simulink model "CubeSatTEST"  (R2024b)
settings: Solver=ode4  StartTime=simul.t0  StopTime=simul.tf  FixedStep=0.01  RelTol=1e-3
values from neighbouring files (symbols this model uses):
  alpha1 = 0.7    [mainSimTEST.m]
  alpha2 = 0.3    [mainSimTEST.m]
undefined symbols (not defined in the file or in its folder): act, DiscIntNeverNeededParam, env, flag, IC, K, orb, sat, sens
libraries: matrix_library x55, simulink_extras x5, simulink x2
(part 8 of 10)

== system CubeSatTEST/Real World/Hardware Models/Actuators/CMG + Control Logic/CMG/State/B assembler ==
  beta : Inport
  delta : Inport  Port=2
  Cos : Trigonometry  Operator=cos
  Cos1 : Trigonometry  Operator=cos
  Gain{,1..3} (4 alike) : Gain  Gain=-1
  Matrix Concatenate : Concatenate  NumInputs=4  Mode=Multidimensional array  ConcatenateDimension=2
  Matrix Concatenate{1..4} (4 alike) : Concatenate  NumInputs=3  Mode=Multidimensional array
  Product{,1..7} (8 alike) : Product
  Selector : Selector  InputPortWidth=4  IndexOptions=Index vector (dialog)  Indices=1  OutputSizes=1
  Selector1 : Selector  InputPortWidth=4  IndexOptions=Index vector (dialog)  Indices=1  OutputSizes=1
  Selector10 : Selector  InputPortWidth=4  IndexOptions=Index vector (dialog)  Indices=4  OutputSizes=1
  Selector11 : Selector  InputPortWidth=4  IndexOptions=Index vector (dialog)  Indices=4  OutputSizes=1
  Selector2 : Selector  InputPortWidth=4  IndexOptions=Index vector (dialog)  Indices=1  OutputSizes=1
  Selector3 : Selector  InputPortWidth=4  IndexOptions=Index vector (dialog)  Indices=2  OutputSizes=1
  Selector4 : Selector  InputPortWidth=4  IndexOptions=Index vector (dialog)  Indices=2  OutputSizes=1
  Selector5 : Selector  InputPortWidth=4  IndexOptions=Index vector (dialog)  Indices=2  OutputSizes=1
  Selector6 : Selector  InputPortWidth=4  IndexOptions=Index vector (dialog)  Indices=3  OutputSizes=1
  Selector7 : Selector  InputPortWidth=4  IndexOptions=Index vector (dialog)  Indices=3  OutputSizes=1
  Selector8 : Selector  InputPortWidth=4  IndexOptions=Index vector (dialog)  Indices=3  OutputSizes=1
  Selector9 : Selector  InputPortWidth=4  IndexOptions=Index vector (dialog)  Indices=4  OutputSizes=1
  Sin : Trigonometry
  Sin1 : Trigonometry
  B : Outport
  wires:
  Cos/1 -> [cosd]
  Sin/1 -> [sind]
  delta/1 -> Cos/1, Sin/1
  beta/1 -> Sin1/1, Cos1/1
  Sin1/1 -> [sinb]
  Cos1/1 -> [cosb]
  Gain/1 -> Matrix Concatenate1/1
  Gain1/1 -> Matrix Concatenate1/2
  Gain2/1 -> Matrix Concatenate2/2
  Gain3/1 -> Matrix Concatenate4/1
  Matrix Concatenate1/1 -> Matrix Concatenate/1
  Matrix Concatenate2/1 -> Matrix Concatenate/2
  Matrix Concatenate3/1 -> Matrix Concatenate/3
  Matrix Concatenate4/1 -> Matrix Concatenate/4
  Matrix Concatenate/1 -> B/1
  Product/1 -> Gain/1
  Product1/1 -> Matrix Concatenate1/3
  Product2/1 -> Gain2/1
  Product3/1 -> Matrix Concatenate2/3
  Product4/1 -> Matrix Concatenate3/1
  Product5/1 -> Matrix Concatenate3/3
  Product6/1 -> Matrix Concatenate4/2
  Product7/1 -> Matrix Concatenate4/3
  Selector/1 -> Gain1/1
  Selector1/1 -> Product1/2
  Selector2/1 -> Product/2
  Selector3/1 -> Matrix Concatenate2/1
  Selector4/1 -> Product2/1
  Selector5/1 -> Product3/2
  Selector6/1 -> Product5/2
  Selector7/1 -> Matrix Concatenate3/2
  Selector8/1 -> Product4/1
  Selector9/1 -> Gain3/1
  Selector10/1 -> Product6/2
  Selector11/1 -> Product7/2
  [sind] -> Selector/1
  [sind] -> Selector3/1
  [sind] -> Selector7/1
  [sind] -> Selector9/1
  [cosd] -> Selector2/1
  [cosd] -> Selector1/1
  [cosd] -> Selector5/1
  [cosd] -> Selector4/1
  [cosd] -> Selector8/1
  [cosd] -> Selector6/1
  [cosd] -> Selector11/1
  [cosd] -> Selector10/1
  [cosb] -> Product/1
  [cosb] -> Product2/2
  [cosb] -> Product4/2
  [cosb] -> Product6/1
  [sinb] -> Product1/1
  [sinb] -> Product3/1
  [sinb] -> Product5/1
  [sinb] -> Product7/1

== system CubeSatTEST/OBC/Navigation1/Sequential Rotations/Q method/q_opt computing/Det 3x3/Adj 3x3/C11 ==
  In1 : Inport
  22 : Selector  NumberOfDimensions=2  InputPortWidth=3  IndexOptions=Index vector (dialog),Index vector (dialog)  Indices=2,2  OutputSizes=1,1
  23 : Selector  NumberOfDimensions=2  InputPortWidth=3  IndexOptions=Index vector (dialog),Index vector (dialog)  Indices=2,3  OutputSizes=1,1
  32 : Selector  NumberOfDimensions=2  InputPortWidth=3  IndexOptions=Index vector (dialog),Index vector (dialog)  Indices=3,2  OutputSizes=1,1
  33 : Selector  NumberOfDimensions=2  InputPortWidth=3  IndexOptions=Index vector (dialog),Index vector (dialog)  Indices=3,3  OutputSizes=1,1
  Product : Product
  Product1 : Product
  Subtract : Sum  Inputs=+-
  Out1 : Outport
  wires:
  In1/1 -> 32/1, 23/1, 33/1, 22/1
  22/1 -> Product/1
  33/1 -> Product/2
  23/1 -> Product1/1
  32/1 -> Product1/2
  Subtract/1 -> Out1/1
  Product/1 -> Subtract/1
  Product1/1 -> Subtract/2

== system CubeSatTEST/OBC/Navigation1/Sequential Rotations/Q method/q_opt computing/Det 3x3/Adj 3x3/C12 ==
  In1 : Inport
  21 : Selector  NumberOfDimensions=2  InputPortWidth=3  IndexOptions=Index vector (dialog),Index vector (dialog)  Indices=2,1  OutputSizes=1,1
  23 : Selector  NumberOfDimensions=2  InputPortWidth=3  IndexOptions=Index vector (dialog),Index vector (dialog)  Indices=2,3  OutputSizes=1,1
  31 : Selector  NumberOfDimensions=2  InputPortWidth=3  IndexOptions=Index vector (dialog),Index vector (dialog)  Indices=3,1  OutputSizes=1,1
  33 : Selector  NumberOfDimensions=2  InputPortWidth=3  IndexOptions=Index vector (dialog),Index vector (dialog)  Indices=3,3  OutputSizes=1,1
  Gain : Gain  Gain=-1
  Product : Product
  Product1 : Product
  Subtract : Sum  Inputs=+-
  Out1 : Outport
  wires:
  In1/1 -> 23/1, 31/1, 33/1, 21/1
  21/1 -> Product/1
  33/1 -> Product/2
  31/1 -> Product1/1
  23/1 -> Product1/2
  Subtract/1 -> Gain/1
  Product/1 -> Subtract/1
  Product1/1 -> Subtract/2
  Gain/1 -> Out1/1

== system CubeSatTEST/OBC/Navigation1/Sequential Rotations/Q method/q_opt computing/Det 3x3/Adj 3x3/C13 ==
  In1 : Inport
  21 : Selector  NumberOfDimensions=2  InputPortWidth=3  IndexOptions=Index vector (dialog),Index vector (dialog)  Indices=2,1  OutputSizes=1,1
  22 : Selector  NumberOfDimensions=2  InputPortWidth=3  IndexOptions=Index vector (dialog),Index vector (dialog)  Indices=2,2  OutputSizes=1,1
  31 : Selector  NumberOfDimensions=2  InputPortWidth=3  IndexOptions=Index vector (dialog),Index vector (dialog)  Indices=3,1  OutputSizes=1,1
  32 : Selector  NumberOfDimensions=2  InputPortWidth=3  IndexOptions=Index vector (dialog),Index vector (dialog)  Indices=3,2  OutputSizes=1,1
  Product : Product
  Product1 : Product
  Subtract : Sum  Inputs=+-
  Out1 : Outport
  wires:
  In1/1 -> 31/1, 22/1, 32/1, 21/1
  21/1 -> Product/1
  32/1 -> Product/2
  22/1 -> Product1/1
  31/1 -> Product1/2
  Subtract/1 -> Out1/1
  Product/1 -> Subtract/1
  Product1/1 -> Subtract/2

== system CubeSatTEST/OBC/Navigation1/Sequential Rotations/Q method/q_opt computing/Det 3x3/Adj 3x3/C21 ==
  In1 : Inport
  12 : Selector  NumberOfDimensions=2  InputPortWidth=3  IndexOptions=Index vector (dialog),Index vector (dialog)  Indices=1,2  OutputSizes=1,1
  13 : Selector  NumberOfDimensions=2  InputPortWidth=3  IndexOptions=Index vector (dialog),Index vector (dialog)  Indices=1,3  OutputSizes=1,1
  32 : Selector  NumberOfDimensions=2  InputPortWidth=3  IndexOptions=Index vector (dialog),Index vector (dialog)  Indices=3,2  OutputSizes=1,1
  33 : Selector  NumberOfDimensions=2  InputPortWidth=3  IndexOptions=Index vector (dialog),Index vector (dialog)  Indices=3,3  OutputSizes=1,1
  Gain : Gain  Gain=-1
  Product : Product
  Product1 : Product
  Subtract : Sum  Inputs=+-
  Out1 : Outport
  wires:
  In1/1 -> 32/1, 13/1, 33/1, 12/1
  12/1 -> Product/1
  33/1 -> Product/2
  13/1 -> Product1/1
  32/1 -> Product1/2
  Subtract/1 -> Gain/1
  Product/1 -> Subtract/1
  Product1/1 -> Subtract/2
  Gain/1 -> Out1/1

== system CubeSatTEST/OBC/Navigation1/Sequential Rotations/Q method/q_opt computing/Det 3x3/Adj 3x3/C22 ==
  In1 : Inport
  11 : Selector  NumberOfDimensions=2  InputPortWidth=3  IndexOptions=Index vector (dialog),Index vector (dialog)  Indices=1,1  OutputSizes=1,1
  13 : Selector  NumberOfDimensions=2  InputPortWidth=3  IndexOptions=Index vector (dialog),Index vector (dialog)  Indices=1,3  OutputSizes=1,1
  31 : Selector  NumberOfDimensions=2  InputPortWidth=3  IndexOptions=Index vector (dialog),Index vector (dialog)  Indices=3,1  OutputSizes=1,1
  33 : Selector  NumberOfDimensions=2  InputPortWidth=3  IndexOptions=Index vector (dialog),Index vector (dialog)  Indices=3,3  OutputSizes=1,1
  Product : Product
  Product1 : Product
  Subtract : Sum  Inputs=+-
  Out1 : Outport
  wires:
  In1/1 -> 31/1, 13/1, 33/1, 11/1
  11/1 -> Product/1
  33/1 -> Product/2
  13/1 -> Product1/1
  31/1 -> Product1/2
  Subtract/1 -> Out1/1
  Product/1 -> Subtract/1
  Product1/1 -> Subtract/2

== system CubeSatTEST/OBC/Navigation1/Sequential Rotations/Q method/q_opt computing/Det 3x3/Adj 3x3/C23 ==
  In1 : Inport
  11 : Selector  NumberOfDimensions=2  InputPortWidth=3  IndexOptions=Index vector (dialog),Index vector (dialog)  Indices=1,1  OutputSizes=1,1
  12 : Selector  NumberOfDimensions=2  InputPortWidth=3  IndexOptions=Index vector (dialog),Index vector (dialog)  Indices=1,2  OutputSizes=1,1
  31 : Selector  NumberOfDimensions=2  InputPortWidth=3  IndexOptions=Index vector (dialog),Index vector (dialog)  Indices=3,1  OutputSizes=1,1
  32 : Selector  NumberOfDimensions=2  InputPortWidth=3  IndexOptions=Index vector (dialog),Index vector (dialog)  Indices=3,2  OutputSizes=1,1
  Gain : Gain  Gain=-1
  Product : Product
  Product1 : Product
  Subtract : Sum  Inputs=+-
  Out1 : Outport
  wires:
  In1/1 -> 12/1, 31/1, 32/1, 11/1
  11/1 -> Product/1
  32/1 -> Product/2
  31/1 -> Product1/1
  12/1 -> Product1/2
  Subtract/1 -> Gain/1
  Product/1 -> Subtract/1
  Product1/1 -> Subtract/2
  Gain/1 -> Out1/1

== system CubeSatTEST/OBC/Navigation1/Sequential Rotations/Q method/q_opt computing/Det 3x3/Adj 3x3/C31 ==
  In1 : Inport
  12 : Selector  NumberOfDimensions=2  InputPortWidth=3  IndexOptions=Index vector (dialog),Index vector (dialog)  Indices=1,2  OutputSizes=1,1
  13 : Selector  NumberOfDimensions=2  InputPortWidth=3  IndexOptions=Index vector (dialog),Index vector (dialog)  Indices=1,3  OutputSizes=1,1
  22 : Selector  NumberOfDimensions=2  InputPortWidth=3  IndexOptions=Index vector (dialog),Index vector (dialog)  Indices=2,2  OutputSizes=1,1
  23 : Selector  NumberOfDimensions=2  InputPortWidth=3  IndexOptions=Index vector (dialog),Index vector (dialog)  Indices=2,3  OutputSizes=1,1
  Product : Product
  Product1 : Product
  Subtract : Sum  Inputs=+-
  Out1 : Outport
  wires:
  In1/1 -> 22/1, 13/1, 23/1, 12/1
  12/1 -> Product/1
  23/1 -> Product/2
  13/1 -> Product1/1
  22/1 -> Product1/2
  Subtract/1 -> Out1/1
  Product/1 -> Subtract/1
  Product1/1 -> Subtract/2

== system CubeSatTEST/OBC/Navigation1/Sequential Rotations/Q method/q_opt computing/Det 3x3/Adj 3x3/C32 ==
  In1 : Inport
  11 : Selector  NumberOfDimensions=2  InputPortWidth=3  IndexOptions=Index vector (dialog),Index vector (dialog)  Indices=1,1  OutputSizes=1,1
  13 : Selector  NumberOfDimensions=2  InputPortWidth=3  IndexOptions=Index vector (dialog),Index vector (dialog)  Indices=1,3  OutputSizes=1,1
  23 : Selector  NumberOfDimensions=2  InputPortWidth=3  IndexOptions=Index vector (dialog),Index vector (dialog)  Indices=2,3  OutputSizes=1,1
  31 : Selector  NumberOfDimensions=2  InputPortWidth=3  IndexOptions=Index vector (dialog),Index vector (dialog)  Indices=3,1  OutputSizes=1,1
  Gain : Gain  Gain=-1
  Product : Product
  Product1 : Product
  Subtract : Sum  Inputs=+-
  Out1 : Outport
  wires:
  In1/1 -> 31/1, 13/1, 23/1, 11/1
  11/1 -> Product/1
  23/1 -> Product/2
  13/1 -> Product1/1
  31/1 -> Product1/2
  Subtract/1 -> Gain/1
  Product/1 -> Subtract/1
  Product1/1 -> Subtract/2
  Gain/1 -> Out1/1

== system CubeSatTEST/OBC/Navigation1/Sequential Rotations/Q method/q_opt computing/Det 3x3/Adj 3x3/C33 ==
  In1 : Inport
  11 : Selector  NumberOfDimensions=2  InputPortWidth=3  IndexOptions=Index vector (dialog),Index vector (dialog)  Indices=1,1  OutputSizes=1,1
  12 : Selector  NumberOfDimensions=2  InputPortWidth=3  IndexOptions=Index vector (dialog),Index vector (dialog)  Indices=1,2  OutputSizes=1,1
  21 : Selector  NumberOfDimensions=2  InputPortWidth=3  IndexOptions=Index vector (dialog),Index vector (dialog)  Indices=2,1  OutputSizes=1,1
  22 : Selector  NumberOfDimensions=2  InputPortWidth=3  IndexOptions=Index vector (dialog),Index vector (dialog)  Indices=2,2  OutputSizes=1,1
  Product : Product
  Product1 : Product
  Subtract : Sum  Inputs=+-
  Out1 : Outport
  wires:
  In1/1 -> 21/1, 12/1, 22/1, 11/1
  11/1 -> Product/1
  22/1 -> Product/2
  12/1 -> Product1/1
  21/1 -> Product1/2
  Subtract/1 -> Out1/1
  Product/1 -> Subtract/1
  Product1/1 -> Subtract/2

== system CubeSatTEST/OBC/Navigation1/Sequential Rotations/Q method/q_opt computing/||q||1/[q (x)]/Psi(q) ==
  In1 : Inport
  Demux : Demux
  Gain{,1..5} (6 alike) : Gain  Gain=-1
  Matrix Concatenate : Concatenate  NumInputs=3  Mode=Multidimensional array  ConcatenateDimension=2
  Matrix Concatenate1 : Concatenate  NumInputs=4  Mode=Multidimensional array
  Matrix Concatenate2 : Concatenate  NumInputs=4  Mode=Multidimensional array
  Matrix Concatenate3 : Concatenate  NumInputs=4  Mode=Multidimensional array
  Out1 : Outport
  wires:
  [q1] -> Matrix Concatenate3/2
  [q1] -> Gain2/1
  [q1] -> Gain/1
  [q2] -> Gain4/1
  [q2] -> Gain1/1
  [q2] -> Matrix Concatenate1/3
  [q3] -> Gain5/1
  [q3] -> Matrix Concatenate2/1
  [q3] -> Gain3/1
  [q4] -> Matrix Concatenate3/3
  [q4] -> Matrix Concatenate2/2
  [q4] -> Matrix Concatenate1/1
  Gain5/1 -> Matrix Concatenate3/4
  Gain4/1 -> Matrix Concatenate3/1
  Gain3/1 -> Matrix Concatenate1/2
  Gain/1 -> Matrix Concatenate1/4
  Gain2/1 -> Matrix Concatenate2/3
  Gain1/1 -> Matrix Concatenate2/4
  Matrix Concatenate3/1 -> Matrix Concatenate/3
  Matrix Concatenate2/1 -> Matrix Concatenate/2
  Matrix Concatenate1/1 -> Matrix Concatenate/1
  Matrix Concatenate/1 -> Out1/1
  Demux/1 -> [q1]
  Demux/4 -> [q4]
  Demux/3 -> [q3]
  Demux/2 -> [q2]
  In1/1 -> Demux/1

== system CubeSatTEST/OBC/Navigation1/Sequential Rotations + Q method/Q method/q_opt computing/Det 3x3/Adj 3x3/C11 ==
  In1 : Inport
  22 : Selector  NumberOfDimensions=2  InputPortWidth=3  IndexOptions=Index vector (dialog),Index vector (dialog)  Indices=2,2  OutputSizes=1,1
  23 : Selector  NumberOfDimensions=2  InputPortWidth=3  IndexOptions=Index vector (dialog),Index vector (dialog)  Indices=2,3  OutputSizes=1,1
  32 : Selector  NumberOfDimensions=2  InputPortWidth=3  IndexOptions=Index vector (dialog),Index vector (dialog)  Indices=3,2  OutputSizes=1,1
  33 : Selector  NumberOfDimensions=2  InputPortWidth=3  IndexOptions=Index vector (dialog),Index vector (dialog)  Indices=3,3  OutputSizes=1,1
  Product : Product
  Product1 : Product
  Subtract : Sum  Inputs=+-
  Out1 : Outport
  wires:
  In1/1 -> 32/1, 23/1, 33/1, 22/1
  22/1 -> Product/1
  33/1 -> Product/2
  23/1 -> Product1/1
  32/1 -> Product1/2
  Subtract/1 -> Out1/1
  Product/1 -> Subtract/1
  Product1/1 -> Subtract/2

== system CubeSatTEST/OBC/Navigation1/Sequential Rotations + Q method/Q method/q_opt computing/Det 3x3/Adj 3x3/C12 ==
  In1 : Inport
  21 : Selector  NumberOfDimensions=2  InputPortWidth=3  IndexOptions=Index vector (dialog),Index vector (dialog)  Indices=2,1  OutputSizes=1,1
  23 : Selector  NumberOfDimensions=2  InputPortWidth=3  IndexOptions=Index vector (dialog),Index vector (dialog)  Indices=2,3  OutputSizes=1,1
  31 : Selector  NumberOfDimensions=2  InputPortWidth=3  IndexOptions=Index vector (dialog),Index vector (dialog)  Indices=3,1  OutputSizes=1,1
  33 : Selector  NumberOfDimensions=2  InputPortWidth=3  IndexOptions=Index vector (dialog),Index vector (dialog)  Indices=3,3  OutputSizes=1,1
  Gain : Gain  Gain=-1
  Product : Product
  Product1 : Product
  Subtract : Sum  Inputs=+-
  Out1 : Outport
  wires:
  In1/1 -> 23/1, 31/1, 33/1, 21/1
  21/1 -> Product/1
  33/1 -> Product/2
  31/1 -> Product1/1
  23/1 -> Product1/2
  Subtract/1 -> Gain/1
  Product/1 -> Subtract/1
  Product1/1 -> Subtract/2
  Gain/1 -> Out1/1

== system CubeSatTEST/OBC/Navigation1/Sequential Rotations + Q method/Q method/q_opt computing/Det 3x3/Adj 3x3/C13 ==
  In1 : Inport
  21 : Selector  NumberOfDimensions=2  InputPortWidth=3  IndexOptions=Index vector (dialog),Index vector (dialog)  Indices=2,1  OutputSizes=1,1
  22 : Selector  NumberOfDimensions=2  InputPortWidth=3  IndexOptions=Index vector (dialog),Index vector (dialog)  Indices=2,2  OutputSizes=1,1
  31 : Selector  NumberOfDimensions=2  InputPortWidth=3  IndexOptions=Index vector (dialog),Index vector (dialog)  Indices=3,1  OutputSizes=1,1
  32 : Selector  NumberOfDimensions=2  InputPortWidth=3  IndexOptions=Index vector (dialog),Index vector (dialog)  Indices=3,2  OutputSizes=1,1
  Product : Product
  Product1 : Product
  Subtract : Sum  Inputs=+-
  Out1 : Outport
  wires:
  In1/1 -> 31/1, 22/1, 32/1, 21/1
  21/1 -> Product/1
  32/1 -> Product/2
  22/1 -> Product1/1
  31/1 -> Product1/2
  Subtract/1 -> Out1/1
  Product/1 -> Subtract/1
  Product1/1 -> Subtract/2

== system CubeSatTEST/OBC/Navigation1/Sequential Rotations + Q method/Q method/q_opt computing/Det 3x3/Adj 3x3/C21 ==
  In1 : Inport
  12 : Selector  NumberOfDimensions=2  InputPortWidth=3  IndexOptions=Index vector (dialog),Index vector (dialog)  Indices=1,2  OutputSizes=1,1
  13 : Selector  NumberOfDimensions=2  InputPortWidth=3  IndexOptions=Index vector (dialog),Index vector (dialog)  Indices=1,3  OutputSizes=1,1
  32 : Selector  NumberOfDimensions=2  InputPortWidth=3  IndexOptions=Index vector (dialog),Index vector (dialog)  Indices=3,2  OutputSizes=1,1
  33 : Selector  NumberOfDimensions=2  InputPortWidth=3  IndexOptions=Index vector (dialog),Index vector (dialog)  Indices=3,3  OutputSizes=1,1
  Gain : Gain  Gain=-1
  Product : Product
  Product1 : Product
  Subtract : Sum  Inputs=+-
  Out1 : Outport
  wires:
  In1/1 -> 32/1, 13/1, 33/1, 12/1
  12/1 -> Product/1
  33/1 -> Product/2
  13/1 -> Product1/1
  32/1 -> Product1/2
  Subtract/1 -> Gain/1
  Product/1 -> Subtract/1
  Product1/1 -> Subtract/2
  Gain/1 -> Out1/1

== system CubeSatTEST/OBC/Navigation1/Sequential Rotations + Q method/Q method/q_opt computing/Det 3x3/Adj 3x3/C22 ==
  In1 : Inport
  11 : Selector  NumberOfDimensions=2  InputPortWidth=3  IndexOptions=Index vector (dialog),Index vector (dialog)  Indices=1,1  OutputSizes=1,1
  13 : Selector  NumberOfDimensions=2  InputPortWidth=3  IndexOptions=Index vector (dialog),Index vector (dialog)  Indices=1,3  OutputSizes=1,1
  31 : Selector  NumberOfDimensions=2  InputPortWidth=3  IndexOptions=Index vector (dialog),Index vector (dialog)  Indices=3,1  OutputSizes=1,1
  33 : Selector  NumberOfDimensions=2  InputPortWidth=3  IndexOptions=Index vector (dialog),Index vector (dialog)  Indices=3,3  OutputSizes=1,1
  Product : Product
  Product1 : Product
  Subtract : Sum  Inputs=+-
  Out1 : Outport
  wires:
  In1/1 -> 31/1, 13/1, 33/1, 11/1
  11/1 -> Product/1
  33/1 -> Product/2
  13/1 -> Product1/1
  31/1 -> Product1/2
  Subtract/1 -> Out1/1
  Product/1 -> Subtract/1
  Product1/1 -> Subtract/2

== system CubeSatTEST/OBC/Navigation1/Sequential Rotations + Q method/Q method/q_opt computing/Det 3x3/Adj 3x3/C23 ==
  In1 : Inport
  11 : Selector  NumberOfDimensions=2  InputPortWidth=3  IndexOptions=Index vector (dialog),Index vector (dialog)  Indices=1,1  OutputSizes=1,1
  12 : Selector  NumberOfDimensions=2  InputPortWidth=3  IndexOptions=Index vector (dialog),Index vector (dialog)  Indices=1,2  OutputSizes=1,1
  31 : Selector  NumberOfDimensions=2  InputPortWidth=3  IndexOptions=Index vector (dialog),Index vector (dialog)  Indices=3,1  OutputSizes=1,1
  32 : Selector  NumberOfDimensions=2  InputPortWidth=3  IndexOptions=Index vector (dialog),Index vector (dialog)  Indices=3,2  OutputSizes=1,1
  Gain : Gain  Gain=-1
  Product : Product
  Product1 : Product
  Subtract : Sum  Inputs=+-
  Out1 : Outport
  wires:
  In1/1 -> 12/1, 31/1, 32/1, 11/1
  11/1 -> Product/1
  32/1 -> Product/2
  31/1 -> Product1/1
  12/1 -> Product1/2
  Subtract/1 -> Gain/1
  Product/1 -> Subtract/1
  Product1/1 -> Subtract/2
  Gain/1 -> Out1/1

== system CubeSatTEST/OBC/Navigation1/Sequential Rotations + Q method/Q method/q_opt computing/Det 3x3/Adj 3x3/C31 ==
  In1 : Inport
  12 : Selector  NumberOfDimensions=2  InputPortWidth=3  IndexOptions=Index vector (dialog),Index vector (dialog)  Indices=1,2  OutputSizes=1,1
  13 : Selector  NumberOfDimensions=2  InputPortWidth=3  IndexOptions=Index vector (dialog),Index vector (dialog)  Indices=1,3  OutputSizes=1,1
  22 : Selector  NumberOfDimensions=2  InputPortWidth=3  IndexOptions=Index vector (dialog),Index vector (dialog)  Indices=2,2  OutputSizes=1,1
  23 : Selector  NumberOfDimensions=2  InputPortWidth=3  IndexOptions=Index vector (dialog),Index vector (dialog)  Indices=2,3  OutputSizes=1,1
  Product : Product
  Product1 : Product
  Subtract : Sum  Inputs=+-
  Out1 : Outport
  wires:
  In1/1 -> 22/1, 13/1, 23/1, 12/1
  12/1 -> Product/1
  23/1 -> Product/2
  13/1 -> Product1/1
  22/1 -> Product1/2
  Subtract/1 -> Out1/1
  Product/1 -> Subtract/1
  Product1/1 -> Subtract/2

== system CubeSatTEST/OBC/Navigation1/Sequential Rotations + Q method/Q method/q_opt computing/Det 3x3/Adj 3x3/C32 ==
  In1 : Inport
  11 : Selector  NumberOfDimensions=2  InputPortWidth=3  IndexOptions=Index vector (dialog),Index vector (dialog)  Indices=1,1  OutputSizes=1,1
  13 : Selector  NumberOfDimensions=2  InputPortWidth=3  IndexOptions=Index vector (dialog),Index vector (dialog)  Indices=1,3  OutputSizes=1,1
  23 : Selector  NumberOfDimensions=2  InputPortWidth=3  IndexOptions=Index vector (dialog),Index vector (dialog)  Indices=2,3  OutputSizes=1,1
  31 : Selector  NumberOfDimensions=2  InputPortWidth=3  IndexOptions=Index vector (dialog),Index vector (dialog)  Indices=3,1  OutputSizes=1,1
  Gain : Gain  Gain=-1
  Product : Product
  Product1 : Product
  Subtract : Sum  Inputs=+-
  Out1 : Outport
  wires:
  In1/1 -> 31/1, 13/1, 23/1, 11/1
  11/1 -> Product/1
  23/1 -> Product/2
  13/1 -> Product1/1
  31/1 -> Product1/2
  Subtract/1 -> Gain/1
  Product/1 -> Subtract/1
  Product1/1 -> Subtract/2
  Gain/1 -> Out1/1

== system CubeSatTEST/OBC/Navigation1/Sequential Rotations + Q method/Q method/q_opt computing/Det 3x3/Adj 3x3/C33 ==
  In1 : Inport
  11 : Selector  NumberOfDimensions=2  InputPortWidth=3  IndexOptions=Index vector (dialog),Index vector (dialog)  Indices=1,1  OutputSizes=1,1
  12 : Selector  NumberOfDimensions=2  InputPortWidth=3  IndexOptions=Index vector (dialog),Index vector (dialog)  Indices=1,2  OutputSizes=1,1
  21 : Selector  NumberOfDimensions=2  InputPortWidth=3  IndexOptions=Index vector (dialog),Index vector (dialog)  Indices=2,1  OutputSizes=1,1
  22 : Selector  NumberOfDimensions=2  InputPortWidth=3  IndexOptions=Index vector (dialog),Index vector (dialog)  Indices=2,2  OutputSizes=1,1
  Product : Product
  Product1 : Product
  Subtract : Sum  Inputs=+-
  Out1 : Outport
  wires:
  In1/1 -> 21/1, 12/1, 22/1, 11/1
  11/1 -> Product/1
  22/1 -> Product/2
  12/1 -> Product1/1
  21/1 -> Product1/2
  Subtract/1 -> Out1/1
  Product/1 -> Subtract/1
  Product1/1 -> Subtract/2

== system CubeSatTEST/OBC/Navigation1/Sequential Rotations + Q method/Q method/q_opt computing/||q||1/[q (x)]/Psi(q) ==
  In1 : Inport
  Demux : Demux
  Gain{,1..5} (6 alike) : Gain  Gain=-1
  Matrix Concatenate : Concatenate  NumInputs=3  Mode=Multidimensional array  ConcatenateDimension=2
  Matrix Concatenate1 : Concatenate  NumInputs=4  Mode=Multidimensional array
  Matrix Concatenate2 : Concatenate  NumInputs=4  Mode=Multidimensional array
  Matrix Concatenate3 : Concatenate  NumInputs=4  Mode=Multidimensional array
  Out1 : Outport
  wires:
  [q1] -> Matrix Concatenate3/2
  [q1] -> Gain2/1
  [q1] -> Gain/1
  [q2] -> Gain4/1
  [q2] -> Gain1/1
  [q2] -> Matrix Concatenate1/3
  [q3] -> Gain5/1
  [q3] -> Matrix Concatenate2/1
  [q3] -> Gain3/1
  [q4] -> Matrix Concatenate3/3
  [q4] -> Matrix Concatenate2/2
  [q4] -> Matrix Concatenate1/1
  Gain5/1 -> Matrix Concatenate3/4
  Gain4/1 -> Matrix Concatenate3/1
  Gain3/1 -> Matrix Concatenate1/2
  Gain/1 -> Matrix Concatenate1/4
  Gain2/1 -> Matrix Concatenate2/3
  Gain1/1 -> Matrix Concatenate2/4
  Matrix Concatenate3/1 -> Matrix Concatenate/3
  Matrix Concatenate2/1 -> Matrix Concatenate/2
  Matrix Concatenate1/1 -> Matrix Concatenate/1
  Matrix Concatenate/1 -> Out1/1
  Demux/1 -> [q1]
  Demux/4 -> [q4]
  Demux/3 -> [q3]
  Demux/2 -> [q2]
  In1/1 -> Demux/1

== system CubeSatTEST/OBC/Navigation1/Sequential Rotations + Q method/Z/Q method z/q_opt computing/Adj 3x3/C11 ==
  In1 : Inport
  22 : Selector  NumberOfDimensions=2  InputPortWidth=3  IndexOptions=Index vector (dialog),Index vector (dialog)  Indices=2,2  OutputSizes=1,1
  23 : Selector  NumberOfDimensions=2  InputPortWidth=3  IndexOptions=Index vector (dialog),Index vector (dialog)  Indices=2,3  OutputSizes=1,1
  32 : Selector  NumberOfDimensions=2  InputPortWidth=3  IndexOptions=Index vector (dialog),Index vector (dialog)  Indices=3,2  OutputSizes=1,1
  33 : Selector  NumberOfDimensions=2  InputPortWidth=3  IndexOptions=Index vector (dialog),Index vector (dialog)  Indices=3,3  OutputSizes=1,1
  Product : Product
  Product1 : Product
  Subtract : Sum  Inputs=+-
  Out1 : Outport
  wires:
  In1/1 -> 32/1, 23/1, 33/1, 22/1
  22/1 -> Product/1
  33/1 -> Product/2
  23/1 -> Product1/1
  32/1 -> Product1/2
  Subtract/1 -> Out1/1
  Product/1 -> Subtract/1
  Product1/1 -> Subtract/2

== system CubeSatTEST/OBC/Navigation1/Sequential Rotations + Q method/Z/Q method z/q_opt computing/Adj 3x3/C12 ==
  In1 : Inport
  21 : Selector  NumberOfDimensions=2  InputPortWidth=3  IndexOptions=Index vector (dialog),Index vector (dialog)  Indices=2,1  OutputSizes=1,1
  23 : Selector  NumberOfDimensions=2  InputPortWidth=3  IndexOptions=Index vector (dialog),Index vector (dialog)  Indices=2,3  OutputSizes=1,1
  31 : Selector  NumberOfDimensions=2  InputPortWidth=3  IndexOptions=Index vector (dialog),Index vector (dialog)  Indices=3,1  OutputSizes=1,1
  33 : Selector  NumberOfDimensions=2  InputPortWidth=3  IndexOptions=Index vector (dialog),Index vector (dialog)  Indices=3,3  OutputSizes=1,1
  Gain : Gain  Gain=-1
  Product : Product
  Product1 : Product
  Subtract : Sum  Inputs=+-
  Out1 : Outport
  wires:
  In1/1 -> 23/1, 31/1, 33/1, 21/1
  21/1 -> Product/1
  33/1 -> Product/2
  31/1 -> Product1/1
  23/1 -> Product1/2
  Subtract/1 -> Gain/1
  Product/1 -> Subtract/1
  Product1/1 -> Subtract/2
  Gain/1 -> Out1/1

== system CubeSatTEST/OBC/Navigation1/Sequential Rotations + Q method/Z/Q method z/q_opt computing/Adj 3x3/C13 ==
  In1 : Inport
  21 : Selector  NumberOfDimensions=2  InputPortWidth=3  IndexOptions=Index vector (dialog),Index vector (dialog)  Indices=2,1  OutputSizes=1,1
  22 : Selector  NumberOfDimensions=2  InputPortWidth=3  IndexOptions=Index vector (dialog),Index vector (dialog)  Indices=2,2  OutputSizes=1,1
  31 : Selector  NumberOfDimensions=2  InputPortWidth=3  IndexOptions=Index vector (dialog),Index vector (dialog)  Indices=3,1  OutputSizes=1,1
  32 : Selector  NumberOfDimensions=2  InputPortWidth=3  IndexOptions=Index vector (dialog),Index vector (dialog)  Indices=3,2  OutputSizes=1,1
  Product : Product
  Product1 : Product
  Subtract : Sum  Inputs=+-
  Out1 : Outport
  wires:
  In1/1 -> 31/1, 22/1, 32/1, 21/1
  21/1 -> Product/1
  32/1 -> Product/2
  22/1 -> Product1/1
  31/1 -> Product1/2
  Subtract/1 -> Out1/1
  Product/1 -> Subtract/1
  Product1/1 -> Subtract/2

== system CubeSatTEST/OBC/Navigation1/Sequential Rotations + Q method/Z/Q method z/q_opt computing/Adj 3x3/C21 ==
  In1 : Inport
  12 : Selector  NumberOfDimensions=2  InputPortWidth=3  IndexOptions=Index vector (dialog),Index vector (dialog)  Indices=1,2  OutputSizes=1,1
  13 : Selector  NumberOfDimensions=2  InputPortWidth=3  IndexOptions=Index vector (dialog),Index vector (dialog)  Indices=1,3  OutputSizes=1,1
  32 : Selector  NumberOfDimensions=2  InputPortWidth=3  IndexOptions=Index vector (dialog),Index vector (dialog)  Indices=3,2  OutputSizes=1,1
  33 : Selector  NumberOfDimensions=2  InputPortWidth=3  IndexOptions=Index vector (dialog),Index vector (dialog)  Indices=3,3  OutputSizes=1,1
  Gain : Gain  Gain=-1
  Product : Product
  Product1 : Product
  Subtract : Sum  Inputs=+-
  Out1 : Outport
  wires:
  In1/1 -> 32/1, 13/1, 33/1, 12/1
  12/1 -> Product/1
  33/1 -> Product/2
  13/1 -> Product1/1
  32/1 -> Product1/2
  Subtract/1 -> Gain/1
  Product/1 -> Subtract/1
  Product1/1 -> Subtract/2
  Gain/1 -> Out1/1

== system CubeSatTEST/OBC/Navigation1/Sequential Rotations + Q method/Z/Q method z/q_opt computing/Adj 3x3/C22 ==
  In1 : Inport
  11 : Selector  NumberOfDimensions=2  InputPortWidth=3  IndexOptions=Index vector (dialog),Index vector (dialog)  Indices=1,1  OutputSizes=1,1
  13 : Selector  NumberOfDimensions=2  InputPortWidth=3  IndexOptions=Index vector (dialog),Index vector (dialog)  Indices=1,3  OutputSizes=1,1
  31 : Selector  NumberOfDimensions=2  InputPortWidth=3  IndexOptions=Index vector (dialog),Index vector (dialog)  Indices=3,1  OutputSizes=1,1
  33 : Selector  NumberOfDimensions=2  InputPortWidth=3  IndexOptions=Index vector (dialog),Index vector (dialog)  Indices=3,3  OutputSizes=1,1
  Product : Product
  Product1 : Product
  Subtract : Sum  Inputs=+-
  Out1 : Outport
  wires:
  In1/1 -> 31/1, 13/1, 33/1, 11/1
  11/1 -> Product/1
  33/1 -> Product/2
  13/1 -> Product1/1
  31/1 -> Product1/2
  Subtract/1 -> Out1/1
  Product/1 -> Subtract/1
  Product1/1 -> Subtract/2

== system CubeSatTEST/OBC/Navigation1/Sequential Rotations + Q method/Z/Q method z/q_opt computing/Adj 3x3/C23 ==
  In1 : Inport
  11 : Selector  NumberOfDimensions=2  InputPortWidth=3  IndexOptions=Index vector (dialog),Index vector (dialog)  Indices=1,1  OutputSizes=1,1
  12 : Selector  NumberOfDimensions=2  InputPortWidth=3  IndexOptions=Index vector (dialog),Index vector (dialog)  Indices=1,2  OutputSizes=1,1
  31 : Selector  NumberOfDimensions=2  InputPortWidth=3  IndexOptions=Index vector (dialog),Index vector (dialog)  Indices=3,1  OutputSizes=1,1
  32 : Selector  NumberOfDimensions=2  InputPortWidth=3  IndexOptions=Index vector (dialog),Index vector (dialog)  Indices=3,2  OutputSizes=1,1
  Gain : Gain  Gain=-1
  Product : Product
  Product1 : Product
  Subtract : Sum  Inputs=+-
  Out1 : Outport
  wires:
  In1/1 -> 12/1, 31/1, 32/1, 11/1
  11/1 -> Product/1
  32/1 -> Product/2
  31/1 -> Product1/1
  12/1 -> Product1/2
  Subtract/1 -> Gain/1
  Product/1 -> Subtract/1
  Product1/1 -> Subtract/2
  Gain/1 -> Out1/1

== system CubeSatTEST/OBC/Navigation1/Sequential Rotations + Q method/Z/Q method z/q_opt computing/Adj 3x3/C31 ==
  In1 : Inport
  12 : Selector  NumberOfDimensions=2  InputPortWidth=3  IndexOptions=Index vector (dialog),Index vector (dialog)  Indices=1,2  OutputSizes=1,1
  13 : Selector  NumberOfDimensions=2  InputPortWidth=3  IndexOptions=Index vector (dialog),Index vector (dialog)  Indices=1,3  OutputSizes=1,1
  22 : Selector  NumberOfDimensions=2  InputPortWidth=3  IndexOptions=Index vector (dialog),Index vector (dialog)  Indices=2,2  OutputSizes=1,1
  23 : Selector  NumberOfDimensions=2  InputPortWidth=3  IndexOptions=Index vector (dialog),Index vector (dialog)  Indices=2,3  OutputSizes=1,1
  Product : Product
  Product1 : Product
  Subtract : Sum  Inputs=+-
  Out1 : Outport
  wires:
  In1/1 -> 22/1, 13/1, 23/1, 12/1
  12/1 -> Product/1
  23/1 -> Product/2
  13/1 -> Product1/1
  22/1 -> Product1/2
  Subtract/1 -> Out1/1
  Product/1 -> Subtract/1
  Product1/1 -> Subtract/2

== system CubeSatTEST/OBC/Navigation1/Sequential Rotations + Q method/Z/Q method z/q_opt computing/Adj 3x3/C32 ==
  In1 : Inport
  11 : Selector  NumberOfDimensions=2  InputPortWidth=3  IndexOptions=Index vector (dialog),Index vector (dialog)  Indices=1,1  OutputSizes=1,1
  13 : Selector  NumberOfDimensions=2  InputPortWidth=3  IndexOptions=Index vector (dialog),Index vector (dialog)  Indices=1,3  OutputSizes=1,1
  21 : Selector  NumberOfDimensions=2  InputPortWidth=3  IndexOptions=Index vector (dialog),Index vector (dialog)  Indices=2,1  OutputSizes=1,1
  23 : Selector  NumberOfDimensions=2  InputPortWidth=3  IndexOptions=Index vector (dialog),Index vector (dialog)  Indices=2,3  OutputSizes=1,1
  Gain : Gain  Gain=-1
  Product : Product
  Product1 : Product
  Subtract : Sum  Inputs=+-
  Out1 : Outport
  wires:
  In1/1 -> 21/1, 13/1, 23/1, 11/1
  11/1 -> Product/1
  23/1 -> Product/2
  13/1 -> Product1/1
  21/1 -> Product1/2
  Subtract/1 -> Gain/1
  Product/1 -> Subtract/1
  Product1/1 -> Subtract/2
  Gain/1 -> Out1/1

== system CubeSatTEST/OBC/Navigation1/Sequential Rotations + Q method/Z/Q method z/q_opt computing/Adj 3x3/C33 ==
  In1 : Inport
  11 : Selector  NumberOfDimensions=2  InputPortWidth=3  IndexOptions=Index vector (dialog),Index vector (dialog)  Indices=1,1  OutputSizes=1,1
  12 : Selector  NumberOfDimensions=2  InputPortWidth=3  IndexOptions=Index vector (dialog),Index vector (dialog)  Indices=1,2  OutputSizes=1,1
  21 : Selector  NumberOfDimensions=2  InputPortWidth=3  IndexOptions=Index vector (dialog),Index vector (dialog)  Indices=2,1  OutputSizes=1,1
  22 : Selector  NumberOfDimensions=2  InputPortWidth=3  IndexOptions=Index vector (dialog),Index vector (dialog)  Indices=2,2  OutputSizes=1,1
  Product : Product
  Product1 : Product
  Subtract : Sum  Inputs=+-
  Out1 : Outport
  wires:
  In1/1 -> 21/1, 12/1, 22/1, 11/1
  11/1 -> Product/1
  22/1 -> Product/2
  12/1 -> Product1/1
  21/1 -> Product1/2
  Subtract/1 -> Out1/1
  Product/1 -> Subtract/1
  Product1/1 -> Subtract/2

== system CubeSatTEST/OBC/Navigation1/Sequential Rotations + Q method/Z/Q method z/q_opt computing/Det 3x3/Adj 3x3 ==
  In1 : Inport
  C11 : Subsystem
  C12 : Subsystem
  C13 : Subsystem
  C21 : Subsystem
  C22 : Subsystem
  C23 : Subsystem
  C31 : Subsystem
  C32 : Subsystem
  C33 : Subsystem
  From{,1..8} (9 alike) : From
  Goto : Goto
  Matrix Concatenate : Concatenate  NumInputs=3  Mode=Multidimensional array
  Matrix Concatenate1 : Concatenate  NumInputs=3  Mode=Multidimensional array
  Matrix Concatenate2 : Concatenate  NumInputs=3  Mode=Multidimensional array
  Matrix Concatenate3 : Concatenate  NumInputs=3  Mode=Multidimensional array  ConcatenateDimension=2
  Transpose : Math  Operator=transpose
  Out1 : Outport
  wires:
  Transpose/1 -> Out1/1
  In1/1 -> Goto/1
  C11/1(Out1) -> Matrix Concatenate/1
  C21/1(Out1) -> Matrix Concatenate/2
  C31/1(Out1) -> Matrix Concatenate/3
  C22/1(Out1) -> Matrix Concatenate1/2
  C12/1(Out1) -> Matrix Concatenate1/1
  C32/1(Out1) -> Matrix Concatenate1/3
  C23/1(Out1) -> Matrix Concatenate2/2
  C13/1(Out1) -> Matrix Concatenate2/1
  C33/1(Out1) -> Matrix Concatenate2/3
  Matrix Concatenate3/1 -> Transpose/1
  Matrix Concatenate2/1 -> Matrix Concatenate3/3
  Matrix Concatenate1/1 -> Matrix Concatenate3/2
  Matrix Concatenate/1 -> Matrix Concatenate3/1
  From/1 -> C11/1(In1)
  From1/1 -> C21/1(In1)
  From2/1 -> C31/1(In1)
  From3/1 -> C22/1(In1)
  From4/1 -> C32/1(In1)
  From5/1 -> C12/1(In1)
  From6/1 -> C13/1(In1)
  From7/1 -> C23/1(In1)
  From8/1 -> C33/1(In1)

== system CubeSatTEST/OBC/Navigation1/Sequential Rotations + Q method/Z/Q method z/q_opt computing/||q||1/[q (x)] ==
  In1 : Inport
  Matrix Concatenate : Concatenate  Mode=Multidimensional array  ConcatenateDimension=2
  Psi(q) : Subsystem
  Out1 : Outport
  wires:
  Psi(q)/1(Out1) -> Matrix Concatenate/1
  In1/1 -> Matrix Concatenate/2, Psi(q)/1(In1)
  Matrix Concatenate/1 -> Out1/1

== system CubeSatTEST/OBC/Navigation1/Sequential Rotations + Q method/Z/Q method z/q_opt computing/||q||1/q* ==
  note: Evaluate the quaternion coniugate
  q : Inport
  Demux : Demux
  Gain : Gain  Gain=-1
  Gain1 : Gain  Gain=-1
  Gain2 : Gain  Gain=-1
  Mux : Mux
  q* : Outport
  wires:
  Gain2/1 -> Mux/3
  Gain1/1 -> Mux/2
  Gain/1 -> Mux/1
  Demux/3 -> Gain2/1
  Demux/2 -> Gain1/1
  Demux/1 -> Gain/1
  q/1 -> Demux/1
  Demux/4 -> Mux/4
  Mux/1 -> q*/1

== system CubeSatTEST/OBC/Navigation1/Sequential Rotations + Q method/Z/Y/Q method y/S and Z matrix computing/Trace ==
  In1 : Inport
  Extract Diagonal : matrix_library/Extract Diagonal
  Sum of Elements : Sum  Inputs=+
  Out1 : Outport
  wires:
  In1/1 -> Extract Diagonal/1
  Extract Diagonal/1 -> Sum of Elements/1
  Sum of Elements/1 -> Out1/1

== system CubeSatTEST/OBC/Navigation1/Sequential Rotations + Q method/Z/Y/Q method y/Subsystem/Norm1 ==
  Vector : Inport
  Add : Sum  Inputs=+++
  Demux : Demux  Outputs=3
  Sqrt : Sqrt
  Square : Math  Operator=square
  Square1 : Math  Operator=square
  Square2 : Math  Operator=square
  Norm : Outport
  wires:
  Square/1 -> Add/1
  Add/1 -> Sqrt/1
  Demux/3 -> Square1/1
  Square2/1 -> Add/2
  Square1/1 -> Add/3
  Demux/1 -> Square/1
  Demux/2 -> Square2/1
  Vector/1 -> Demux/1
  Sqrt/1 -> Norm/1

== system CubeSatTEST/OBC/Navigation1/Sequential Rotations + Q method/Z/Y/Q method y/Subsystem/Norm2 ==
  Vector : Inport
  Add : Sum  Inputs=+++
  Demux : Demux  Outputs=3
  Sqrt : Sqrt
  Square : Math  Operator=square
  Square1 : Math  Operator=square
  Square2 : Math  Operator=square
  Norm : Outport
  wires:
  Square/1 -> Add/1
  Add/1 -> Sqrt/1
  Demux/3 -> Square1/1
  Square2/1 -> Add/2
  Square1/1 -> Add/3
  Demux/1 -> Square/1
  Demux/2 -> Square2/1
  Vector/1 -> Demux/1
  Sqrt/1 -> Norm/1

== system CubeSatTEST/OBC/Navigation1/Sequential Rotations + Q method/Z/Y/Q method y/q_opt computing/Adj 3x3 ==
  A : Inport
  C11 : Subsystem
  C12 : Subsystem
  C13 : Subsystem
  C21 : Subsystem
  C22 : Subsystem
  C23 : Subsystem
  C31 : Subsystem
  C32 : Subsystem
  C33 : Subsystem
  From{,1..8} (9 alike) : From
  Goto : Goto
  Matrix Concatenate : Concatenate  NumInputs=3  Mode=Multidimensional array
  Matrix Concatenate1 : Concatenate  NumInputs=3  Mode=Multidimensional array
  Matrix Concatenate2 : Concatenate  NumInputs=3  Mode=Multidimensional array
  Matrix Concatenate3 : Concatenate  NumInputs=3  Mode=Multidimensional array  ConcatenateDimension=2
  Transpose : Math  Operator=transpose
  Adj(A) : Outport
  wires:
  Transpose/1 -> Adj(A)/1
  A/1 -> Goto/1
  C11/1(Out1) -> Matrix Concatenate/1
  C21/1(Out1) -> Matrix Concatenate/2
  C31/1(Out1) -> Matrix Concatenate/3
  C22/1(Out1) -> Matrix Concatenate1/2
  C12/1(Out1) -> Matrix Concatenate1/1
  C32/1(Out1) -> Matrix Concatenate1/3
  C23/1(Out1) -> Matrix Concatenate2/2
  C13/1(Out1) -> Matrix Concatenate2/1
  C33/1(Out1) -> Matrix Concatenate2/3
  Matrix Concatenate3/1 -> Transpose/1
  Matrix Concatenate2/1 -> Matrix Concatenate3/3
  Matrix Concatenate1/1 -> Matrix Concatenate3/2
  Matrix Concatenate/1 -> Matrix Concatenate3/1
  From/1 -> C11/1(In1)
  From1/1 -> C21/1(In1)
  From2/1 -> C31/1(In1)
  From3/1 -> C22/1(In1)
  From4/1 -> C32/1(In1)
  From5/1 -> C12/1(In1)
  From6/1 -> C13/1(In1)
  From7/1 -> C23/1(In1)
  From8/1 -> C33/1(In1)

== system CubeSatTEST/OBC/Navigation1/Sequential Rotations + Q method/Z/Y/Q method y/q_opt computing/Det 3x3 ==
  A : Inport
  Adj 3x3 : Subsystem
  Matrix Multiply : Product  Multiplication=Matrix(*)
  Selector : Selector  NumberOfDimensions=2  InputPortWidth=3  IndexOptions=Index vector (dialog),Index vector (dialog)  Indices=1,1  OutputSizes=1,1
  det(A) : Outport
  wires:
  A/1 -> Adj 3x3/1(In1), Matrix Multiply/1
  Adj 3x3/1(Out1) -> Matrix Multiply/2
  Matrix Multiply/1 -> Selector/1
  Selector/1 -> det(A)/1

== system CubeSatTEST/OBC/Navigation1/Sequential Rotations + Q method/Z/Y/Q method y/q_opt computing/Trace ==
  B : Inport
  Extract Diagonal : matrix_library/Extract Diagonal
  Sum of Elements : Sum  Inputs=+
  tr(B) : Outport
  wires:
  B/1 -> Extract Diagonal/1
  Extract Diagonal/1 -> Sum of Elements/1
  Sum of Elements/1 -> tr(B)/1

== system CubeSatTEST/OBC/Navigation1/Sequential Rotations + Q method/Z/Y/Q method y/q_opt computing/||q||1 ==
  q : Inport
  MatrixMultiply : Product  Multiplication=Matrix(*)
  Scope{,1..4} (5 alike) : Scope
  Selector : Selector  InputPortWidth=4  IndexOptions=Index vector (dialog)  Indices=4  OutputSizes=1
  Sqrt : Sqrt
  "[q (x)]" : Subsystem
  q* : Subsystem
  Out1 : Outport
  wires:
  q/1 -> Scope/1, "[q (x)]"/1(In1), q*/1(q)
  q*/1(q*) -> Scope2/1, MatrixMultiply/2
  "[q (x)]"/1(Out1) -> Scope1/1, MatrixMultiply/1
  MatrixMultiply/1 -> Scope3/1, Selector/1
  Selector/1 -> Scope4/1, Sqrt/1
  Sqrt/1 -> Out1/1

== system CubeSatTEST/OBC/Navigation1/Sequential Rotations + Q method/Z/Y/X/Q method x/B computing ==
  Sb : Inport
  SN : Inport  Port=2
  Bb : Inport  Port=3
  BN : Inport  Port=4
  alpha 1 : Inport  Port=5
  alpha 2 : Inport  Port=6
  Add : Sum
  Add1 : Sum
  Add2 : Sum
  Divide : Product  Inputs=*/
  Divide1 : Product  Inputs=/*
  Product : Product  Multiplication=Matrix(*)
  Product1 : Product  Multiplication=Matrix(*)
  Product2 : Product
  Product3 : Product
  Transpose : Math  Operator=transpose
  Transpose1 : Math  Operator=transpose
  B : Outport
  alpha1_normalised : Outport  Port=2
  alpha2_normalised : Outport  Port=3
  wires:
  alpha 1/1 -> [alpha_1]
  alpha 2/1 -> [alpha_2]
  [alpha_1] -> Divide/1, Add/1
  [alpha_2] -> Add/2
  Add/1 -> Divide/2
  Divide/1 -> [alpha_1_normalised]
  [alpha_2] -> Divide1/2, Add1/2
  Divide1/1 -> [alpha_2_normalised]
  [alpha_1] -> Add1/1
  Add1/1 -> Divide1/1
  SN/1 -> [SN]
  Sb/1 -> [Sb]
  Bb/1 -> [Bb]
  BN/1 -> [BN]
  Product/1 -> Add2/1
  Product1/1 -> Add2/2
  Transpose/1 -> Product/2
  [SN] -> Transpose/1
  [BN] -> Transpose1/1
  Add2/1 -> B/1
  Product2/1 -> Product/1
  [alpha_1_normalised] -> Product2/1
  [Sb] -> Product2/2
  Product3/1 -> Product1/1
  [alpha_2_normalised] -> Product3/1
  [Bb] -> Product3/2
  Transpose1/1 -> Product1/2
  [alpha_1_normalised] -> alpha1_normalised/1
  [alpha_2_normalised] -> alpha2_normalised/1

== system CubeSatTEST/OBC/Navigation1/Sequential Rotations + Q method/Z/Y/X/Q method x/S and Z matrix computing ==
  B : Inport
  Add : Sum
  Add1 : Sum  Inputs=+-
  Add2 : Sum  Inputs=+-
  Add3 : Sum  Inputs=+-
  Add4 : Sum  Commented=on  Inputs=+-
  From1 : From  Commented=on  GotoTag=B
  From3 : From  Commented=on  GotoTag=Z
  From4 : From  Commented=on  GotoTag=Sigma
  From5 : From  Commented=on  GotoTag=S
  From6 : From  Commented=on  GotoTag=Z
  From7 : From  Commented=on  GotoTag=Sigma
  Goto2 : Goto  Commented=on  GotoTag=Sigma
  IdentityMatrix : IdentityMatrix  Commented=on
  Matrix Concatenate : Concatenate  Commented=on  NumInputs=4  Mode=Multidimensional array  ConcatenateDimension=2
  Mux : Mux  Inputs=3
  Product : Product  Commented=on
  Selector : Selector  NumberOfDimensions=2  InputPortWidth=3  IndexOptions=Index vector (dialog),Index vector (dialog)  Indices=2,3  OutputSizes=1,1
  Selector1 : Selector  NumberOfDimensions=2  InputPortWidth=3  IndexOptions=Index vector (dialog),Index vector (dialog)  Indices=3,2  OutputSizes=1,1
  Selector2 : Selector  NumberOfDimensions=2  InputPortWidth=3  IndexOptions=Index vector (dialog),Index vector (dialog)  Indices=3,1  OutputSizes=1,1
  Selector3 : Selector  NumberOfDimensions=2  InputPortWidth=3  IndexOptions=Index vector (dialog),Index vector (dialog)  Indices=1,3  OutputSizes=1,1
  Selector4 : Selector  NumberOfDimensions=2  InputPortWidth=3  IndexOptions=Index vector (dialog),Index vector (dialog)  Indices=1,2  OutputSizes=1,1
  Selector5 : Selector  NumberOfDimensions=2  InputPortWidth=3  IndexOptions=Index vector (dialog),Index vector (dialog)  Indices=2,1  OutputSizes=1,1
  Trace : Subsystem  Commented=on
  Transpose : matrix_library/Transpose
  Transpose1 : matrix_library/Transpose  Commented=on
  S : Outport
  Z : Outport  Port=2
  wires:
  [B] -> Add/1, Transpose/1
  Transpose/1 -> Add/2
  Add/1 -> [S]
  B/1 -> [B]
  From1/1 -> Trace/1(In1)
  Trace/1(Out1) -> Goto2/1
  [B] -> Selector/1, Selector1/1, Selector2/1, Selector5/1, Selector4/1, Selector3/1
  Selector/1 -> Add1/1
  Selector1/1 -> Add1/2
  Selector4/1 -> Add3/1
  Selector5/1 -> Add3/2
  Selector3/1 -> Add2/2
  Selector2/1 -> Add2/1
  Add1/1 -> Mux/1
  Add2/1 -> Mux/2
  Add3/1 -> Mux/3
  Mux/1 -> [Z]
  From3/1 -> Matrix Concatenate/2
  From4/1 -> Product/1
  IdentityMatrix/1 -> Product/2
  Product/1 -> Add4/2
  From5/1 -> Add4/1
  Add4/1 -> Matrix Concatenate/1
  Transpose1/1 -> Matrix Concatenate/3
  From6/1 -> Transpose1/1
  From7/1 -> Matrix Concatenate/4
  [S] -> S/1
  [Z] -> Z/1

== system CubeSatTEST/OBC/Navigation1/Sequential Rotations + Q method/Z/Y/X/Q method x/Subsystem ==
  alpha2_normalised : Inport
  alpha1_normalised : Inport  Port=2
  B_b : Inport  Port=3
  B_N : Inport  Port=4
  S_b : Inport  Port=5
  S_N : Inport  Port=6
  Add : Sum
  Add1 : Sum
  Add2 : Sum
  Constant : Constant  Value=2
  Cross Product : matrix_library/Cross Product
  Cross Product1 : matrix_library/Cross Product
  Dot Product : DotProduct  OutDataTypeStr=Inherit: Inherit via internal rule
  Dot Product1 : DotProduct  OutDataTypeStr=Inherit: Inherit via internal rule
  From16 : From
  Goto12 : Goto
  Math Function : Math  Operator=square
  Math Function1 : Math  Operator=square
  Norm1 : Subsystem
  Norm2 : Subsystem
  Product : Product
  Product1 : Product
  Product2 : Product
  Product3 : Product  Inputs=3
  Sqrt : Sqrt
  lambda_max : Outport
  wires:
  Math Function/1 -> Add/1
  Math Function1/1 -> Add/2
  Dot Product/1 -> [dotb1b2]
  Dot Product1/1 -> [dotr1r2]
  [dotr1r2] -> Product/2
  [dotb1b2] -> Product/1
  B_b/1 -> [Bb]
  S_b/1 -> [Sb]
  B_N/1 -> [BN]
  S_N/1 -> [SN]
  [Sb] -> Dot Product/2
  [Bb] -> Dot Product/1
  [SN] -> Dot Product1/2
  [Bb] -> Cross Product1/1
  [Sb] -> Cross Product1/2
  [BN] -> Cross Product/1
  [SN] -> Cross Product/2
  Cross Product1/1 -> Norm1/1(Vector)
  Cross Product/1 -> Norm2/1(Vector)
  [crossb1b2] -> Product1/1
  [crossr1r2] -> Product1/2
  Product1/1 -> Add1/2
  Product/1 -> Add1/1
  alpha2_normalised/1 -> [alpha2_normalised]
  alpha1_normalised/1 -> [alpha1_normalised]
  [alpha1_normalised] -> Math Function/1
  [alpha2_normalised] -> Math Function1/1
  [alpha2_normalised] -> Product3/3
  [alpha1_normalised] -> Product3/2
  Constant/1 -> Product3/1
  Add1/1 -> [C]
  Product3/1 -> [B]
  Add/1 -> Goto12/1
  From16/1 -> Add2/1
  Add2/1 -> Sqrt/1
  Sqrt/1 -> lambda_max/1
  [BN] -> Dot Product1/1
  Norm1/1(Norm) -> [crossb1b2]  "norm_r"
  Norm2/1(Norm) -> [crossr1r2]  "norm_r"
  Product2/1 -> Add2/2
  [B] -> Product2/1
  [C] -> Product2/2

== system CubeSatTEST/OBC/Navigation1/Sequential Rotations + Q method/Z/Y/X/Q method x/q_opt computing ==
  S : Inport
  Z : Inport  Port=2
  lambda_max : Inport  Port=3
  B : Inport  Port=4
  Add : Sum
  Add1 : Sum  Inputs=+-
  Adj 3x3 : Subsystem
  Det 3x3 : Subsystem
  Divide : Product  Inputs=*/
  IdentityMatrix : IdentityMatrix  OutputDimensions=3  SampleTime=-1
  Matrix Concatenate : Concatenate  Mode=Multidimensional array
  Product : Product
  Product1 : Product  Multiplication=Matrix(*)
  Scope : Scope
  Trace : Subsystem
  ||q||1 : Subsystem
  q_opt : Outport
  wires:
  B/1 -> Trace/1(B)
  lambda_max/1 -> Add/2
  Trace/1(tr(B)) -> Add/1
  Add/1 -> [p]
  IdentityMatrix/1 -> Product/2
  [p] -> Product/1
  Product/1 -> [pI3]
  S/1 -> Add1/2
  [pI3] -> Add1/1
  Add1/1 -> Det 3x3/1(A), Adj 3x3/1(A)
  Matrix Concatenate/1 -> [q]
  [q] -> Divide/1
  Divide/1 -> q_opt/1
  Z/1 -> Product1/2
  Product1/1 -> Matrix Concatenate/1
  ||q||1/1(Out1) -> Divide/2
  [q] -> ||q||1/1(q)
  Adj 3x3/1(Adj(A)) -> Product1/1
  Det 3x3/1(det(A)) -> Scope/1, Matrix Concatenate/2

== system CubeSatTEST/OBC/Navigation1/Sequential Rotations Playground/Q method/q_opt computing/Det 3x3/Adj 3x3/C11 ==
  In1 : Inport
  22 : Selector  NumberOfDimensions=2  InputPortWidth=3  IndexOptions=Index vector (dialog),Index vector (dialog)  Indices=2,2  OutputSizes=1,1
  23 : Selector  NumberOfDimensions=2  InputPortWidth=3  IndexOptions=Index vector (dialog),Index vector (dialog)  Indices=2,3  OutputSizes=1,1
  32 : Selector  NumberOfDimensions=2  InputPortWidth=3  IndexOptions=Index vector (dialog),Index vector (dialog)  Indices=3,2  OutputSizes=1,1
  33 : Selector  NumberOfDimensions=2  InputPortWidth=3  IndexOptions=Index vector (dialog),Index vector (dialog)  Indices=3,3  OutputSizes=1,1
  Product : Product
  Product1 : Product
  Subtract : Sum  Inputs=+-
  Out1 : Outport
  wires:
  In1/1 -> 32/1, 23/1, 33/1, 22/1
  22/1 -> Product/1
  33/1 -> Product/2
  23/1 -> Product1/1
  32/1 -> Product1/2
  Subtract/1 -> Out1/1
  Product/1 -> Subtract/1
  Product1/1 -> Subtract/2

== system CubeSatTEST/OBC/Navigation1/Sequential Rotations Playground/Q method/q_opt computing/Det 3x3/Adj 3x3/C12 ==
  In1 : Inport
  21 : Selector  NumberOfDimensions=2  InputPortWidth=3  IndexOptions=Index vector (dialog),Index vector (dialog)  Indices=2,1  OutputSizes=1,1
  23 : Selector  NumberOfDimensions=2  InputPortWidth=3  IndexOptions=Index vector (dialog),Index vector (dialog)  Indices=2,3  OutputSizes=1,1
  31 : Selector  NumberOfDimensions=2  InputPortWidth=3  IndexOptions=Index vector (dialog),Index vector (dialog)  Indices=3,1  OutputSizes=1,1
  33 : Selector  NumberOfDimensions=2  InputPortWidth=3  IndexOptions=Index vector (dialog),Index vector (dialog)  Indices=3,3  OutputSizes=1,1
  Gain : Gain  Gain=-1
  Product : Product
  Product1 : Product
  Subtract : Sum  Inputs=+-
  Out1 : Outport
  wires:
  In1/1 -> 23/1, 31/1, 33/1, 21/1
  21/1 -> Product/1
  33/1 -> Product/2
  31/1 -> Product1/1
  23/1 -> Product1/2
  Subtract/1 -> Gain/1
  Product/1 -> Subtract/1
  Product1/1 -> Subtract/2
  Gain/1 -> Out1/1
